simulink model "xcoilControlDesign"  (R2024a)
settings: Solver=VariableStepAuto  StartTime=0.0  StopTime=20000  FixedStep=0.001  RelTol=1e-3
PreLoadFcn:
  | xcoilParameters.m
values from neighbouring files (symbols this model uses):
  am1 = 0.0232    [xcoilParameters.m]
  am2 = 1.6211e-04    (= 0.00016211)    [xcoilParameters.m]
  ap1 = 1.9163    [xcoilParameters.m]
  ap2 = 0.0176    [xcoilParameters.m]
  bm = entr(1)    [Adaptivefilter.m]    (also in xcoilParameters.m = 1)
  bp = 0.0413    [xcoilParameters.m]
  gamma = entr(2)    [adaptationLaw.m]    (also in xcoilParameters.m = 1e-10)
  km = 1.6211e-04    (= 0.00016211)    [xcoilParameters.m]
  kp = entr(1)    [adaptationLaw.m]    (also in xcoilParameters.m = 1545.8)
  Ts = 1    [myObjectiveFunction.m]    (also in xcoilParameters.m)
settings Model: Creator=b_ant  LastModifiedBy=b_ant
settings DebuggingCC: UnconnectedInputMsg=warning  UnconnectedOutputMsg=warning  UnconnectedLineMsg=warning
settings ModelReferenceCC: EnableRefExpFcnMdlSchedulingChecks=on
settings RTWCC: GPUComputeCapability=3.5  DLArmComputeVersion=19.05

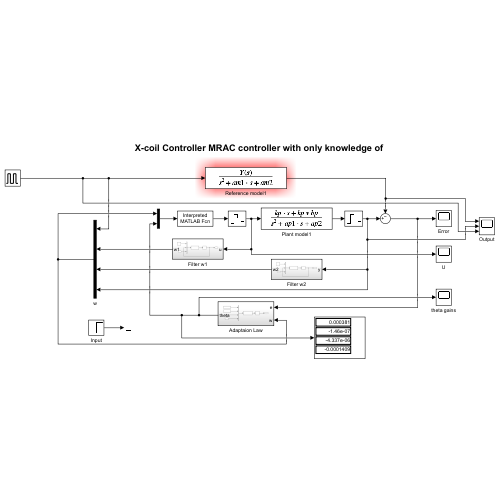
[thumbnail: Simulink's stored preview of the top-level diagram]
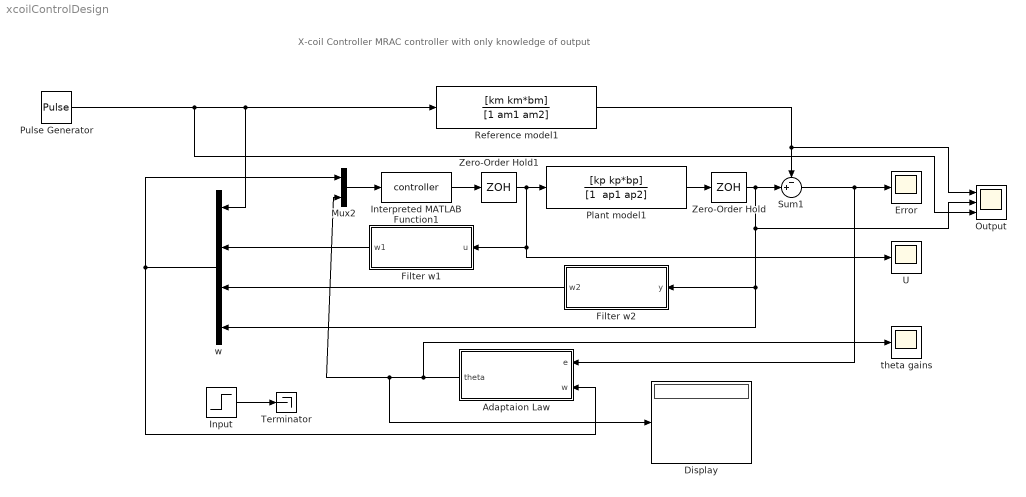
== system xcoilControlDesign ==
  note: X-coil Controller MRAC controller with only knowledge of output
  Adaptaion Law : Subsystem
  Display : Display
  Error : Scope
  Filter w1 : Subsystem
  Filter w2 : Subsystem
  Input : Step  Time=5  Before=1  After=2000  SampleTime=0
  Interpreted MATLAB Function1 : MATLABFcn  MATLABFcn=controller  OutputDimensions=1
  Mux2 : Mux  Inputs=2
  Output : Scope  NumInputPorts=3
  Plant model1 : TransferFcn  Numerator=[kp kp*bp]  Denominator="[1  ap1 ap2]"
  Pulse Generator : DiscretePulseGenerator  PulseType=Time based  Amplitude=2000  Period=5000  PulseWidth=50  PhaseDelay=5
  Reference model1 : TransferFcn  Numerator=[km km*bm]  Denominator=[1 am1 am2]
  Sum1 : Sum  Inputs=-+|
  Terminator : Terminator
  U : Scope
  Zero-Order Hold : ZeroOrderHold  SampleTime=Ts
  Zero-Order Hold1 : ZeroOrderHold  SampleTime=Ts
  theta gains : Scope
  w : Mux
  wires:
  Sum1/1 -> Adaptaion Law/1(e), Error/1
  Reference model1/1 -> Output/1, Sum1/1
  Filter w1/1(w1) -> w/2
  Filter w2/1(w2) -> w/3
  w/1 -> Adaptaion Law/2(w), Mux2/1
  Mux2/1 -> Interpreted MATLAB Function1/1
  Adaptaion Law/1(theta) -> theta gains/1, Display/1, Mux2/2
  Plant model1/1 -> Zero-Order Hold/1
  Zero-Order Hold/1 -> Sum1/2, Filter w2/1(y), w/4, Output/2
  Interpreted MATLAB Function1/1 -> Zero-Order Hold1/1
  Zero-Order Hold1/1 -> U/1, Filter w1/1(u), Plant model1/1
  Input/1 -> Terminator/1
  Pulse Generator/1 -> Output/3, w/1, Reference model1/1

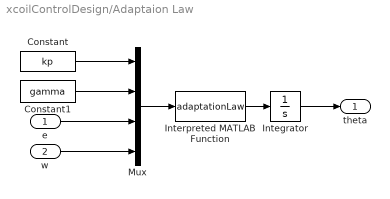
== system xcoilControlDesign/Adaptaion Law ==
  e : Inport
  w : Inport  Port=2
  Constant : Constant  Value=kp
  Constant1 : Constant  Value=gamma
  Integrator : Integrator  InitialCondition=[km/kp,0,0,0]
  Interpreted MATLAB Function : MATLABFcn  MATLABFcn=adaptationLaw  OutputDimensions=4
  Mux : Mux
  theta : Outport
  wires:
  Constant1/1 -> Mux/2
  e/1 -> Mux/3
  w/1 -> Mux/4
  Constant/1 -> Mux/1
  Mux/1 -> Interpreted MATLAB Function/1
  Interpreted MATLAB Function/1 -> Integrator/1
  Integrator/1 -> theta/1

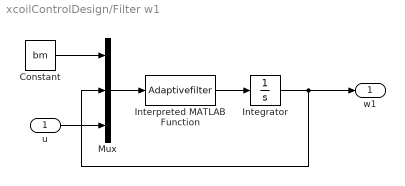
== system xcoilControlDesign/Filter w1 ==
  u : Inport
  Constant : Constant  Value=bm
  Integrator : Integrator  InitialCondition=1
  Interpreted MATLAB Function : MATLABFcn  MATLABFcn=Adaptivefilter  OutputDimensions=1
  Mux : Mux  Inputs=3
  w1 : Outport
  wires:
  u/1 -> Mux/3
  Constant/1 -> Mux/1
  Interpreted MATLAB Function/1 -> Integrator/1
  Mux/1 -> Interpreted MATLAB Function/1
  Integrator/1 -> w1/1, Mux/2

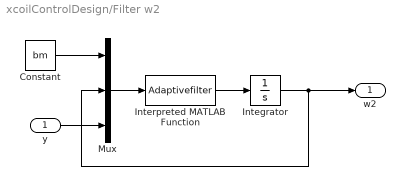
== system xcoilControlDesign/Filter w2 ==
  y : Inport
  Constant : Constant  Value=bm
  Integrator : Integrator  InitialCondition=1
  Interpreted MATLAB Function : MATLABFcn  MATLABFcn=Adaptivefilter  OutputDimensions=1
  Mux : Mux  Inputs=3
  w2 : Outport
  wires:
  y/1 -> Mux/3
  Constant/1 -> Mux/1
  Interpreted MATLAB Function/1 -> Integrator/1
  Mux/1 -> Interpreted MATLAB Function/1
  Integrator/1 -> w2/1, Mux/2
